simulink library "Diamond16AT_UNAL"  (Simulink 7.7)
settings: Solver=ode45  StartTime=0.0  StopTime=10.0  RelTol=1e-3
undefined symbols (not defined in the file or in its folder): Com1, none
libraries: xpcseriallib x2, Diamond16AT_UNAL x2
settings Model: Creator=BolivarNieto  LastModifiedBy=Edgar

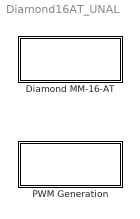
== system Diamond16AT_UNAL ==
  Diamond MM-16-AT : Subsystem
      mask Display: disp('Diamond MM-16-AT')
  PWM Generation : Subsystem
      mask Display: disp('PWM Generation')

== system Diamond16AT_UNAL/Diamond MM-16-AT ==
  MM-16-AT Analog Input : S-Function  FunctionName=addiamondmm16atcustom  Parameters=firstChan, numChans, range, sampleTime, baseDec  EnableBusSupport=off  mask{configuration=16 Single-ended, firstChan=1, numChans=12, range=0 to 5V, sampleTime=0.001, base=300}
      mask prompts: configuration "A/D Configuration"; firstChan "First channel: (From 1 to 8 or 16)"; numChans "Number of channels:"; sampleTime "Sample time:"; base "Base address (HEX):"
      mask help:
      | MM-16-AT
      | Diamond
      | Analog Input
      mask init:
      | phase = 2;
      | [baseDec, maskDisplay, maskDescription] = maskdiamondmm16(phase, configuration, firstChan, numChans, range, base);
      | set_param(gcb, 'MaskDescription', maskDescription);
      | set_param(gcb, 'MaskDisplay', maskDisplay);
      mask StyleString: popup(16 Single-ended|8   Differential inputs),edit,edit,popup(-10V to +10 V|-5V to +5V|-2.5V to +2.5V|-1.25V to +1.25V|-0.625V to +0.625V|0 to 10V|0 to 5V|0 to 2.5V|0 to 1.25V),edit,popup(220 |240 |250 |260 |280 |290 |2A0 |2B0 |2C0 |2D0 |2E0 |300 |330 |340 |350 |360 |380 |390 |3A0 |3C0 |3E0)
      mask Display: disp('MM-16-AT\nDiamond\nAnalog Input'); port_label('output', 1, '1'); port_label('output', 2, '2'); port_label('output', 3, '3'); port_label('output', 4, '4'); port_label('output', 5, '5'); port_label('output', 6, '6'); port_label('output', 7, '7'); port_label('output', 8, '8'); port_label('output', 9, '9'); port_label('output', 10, '10'); port_label('output', 11, '11'); port_label('output', 12, '12');
  MM-16-AT Analog Output : S-Function  FunctionName=dadiamondmm16at_custom  Parameters=channel, range, finalvalue, initValue, sampletime, basedec  EnableBusSupport=off  mask{channel=[ 1 2 3 4], range=0V to 5V, finalValuePop=Set all outputs to 0V, initValue=[0], sampletime=0.001, baseAddress=300}
      mask prompts: channel "Channel vector:"; range "Range vector"; finalValuePop "Behavior at model termination"; initValue "Initial value vector:"; sampletime "Sample time:"; baseAddress "Base address (HEX)"
      mask help:
      | MM-16-AT
      | Diamond Systems
      | Analog Output
      mask init:
      | boardType=1;
      | [maskdisplay, maskdescription, finalvalue, initValue, basedec] = mdadiamondmm16at_custom( boardType, channel, baseAddress, finalValuePop, initValue);
      | set_param(gcb,'MaskDescription',maskdescription);
      | set_param(gcb,'MaskDisplay',maskdisplay);
      mask StyleString: edit,popup(0V to 5V|-5V to 5V),popup(Set all outputs to 0V|Set to last value attained while the model was running),edit,edit,popup(220 |240 |250 |260 |280 |290 |2A0 |2B0 |2C0 |2D0 |2E0 |300 |330 |340 |350 |360 |380 |390 |3A0 |3C0 |3E0)
      mask Display: disp('MM-16-AT\nDiamond\nAnalog Output');port_label('input',1,'1');port_label('input',2,'2');port_label('input',3,'3');port_label('input',4,'4');
  MM-16-AT Digital Output : S-Function  FunctionName=dodiamond16at_custom  Parameters=channel, reset, initValue, sampleTime, basedec  EnableBusSupport=off  mask{channel=[1 2 3 4 5 6 7 8], reset=[0], initValue=[0], sampleTime=0.001, baseAddress2=300}
      mask prompts: channel "Channel vector:"; reset "Reset vector: (0 Hold last value, 1 set to initial value)"; initValue "Initial value vector:"; sampleTime "Sample Time:"; baseAddress2 "Base address (HEX):"
      mask help:
      | MM-16-AT
      | Diamond
      | Digital Output
      mask init:
      | deviceName = 'MM-16-AT';
      | [basedec, maskDisplay, maskDescription, reset, initValue] = mdodiamond16at_custom(deviceName, channel, sampleTime, baseAddress2, reset, initValue);
      | set_param(gcb, 'MaskDisplay', maskDisplay);
      | set_param(gcb, 'MaskDescription', maskDescription);
      mask StyleString: edit,edit,edit,edit,popup(220 |240 |250 |260 |280 |290 |2A0 |2B0 |2C0 |2D0 |2E0 |300 |330 |340 |350 |360 |380 |390 |3A0 |3C0 |3E0)
      mask Display: disp('MM-16-AT\nDiamond\nDigital Output'); port_label('input', 1, '1'); port_label('input', 2, '2'); port_label('input', 3, '3'); port_label('input', 4, '4'); port_label('input', 5, '5'); port_label('input', 6, '6'); port_label('input', 7, '7'); port_label('input', 8, '8');

== system Diamond16AT_UNAL/PWM Generation ==
  Motors - F4  STM - PWM : Subsystem  mask(Protocol for PWM generation through STM-F4){Satura=80, SamTime=0.001}
      mask prompts: Satura "Saturation (%):"; SamTime "Sample Time (s):"
      mask help:
      | Comunication protocol for PWM generation. This block communicates a STM-F4 through serial RS-232 comunication. The STM-F4 generates the PWMs required for motor control.
      |
      | INPUT:  [6x1] Percentage of duty cycle for each of the six motors.
      | OUTPUT: PWM signal to the H-Bridge
      mask Help:
      | Comunication protocol for PWM generation. This block communicates a STM-F4 through serial RS-232 comunication. The STM-F4 generates the PWMs required for motor control.
      | 
      | INPUT:  [6x1] Percentage of duty cycle for each of the six motors.
      | OUTPUT: PWM signal to the H-Bridge
  SG - Digital IO PWM Generation : Subsystem  mask(Stewart Gough Motors Block  ){PWM_amp=4, PWM_freq=1000, Rpm2Pwm=1, SampleTime_ed=0.001}
      mask prompts: PWM_amp "PWM Amplitude"; PWM_freq "PWM frequency (Hz)"; Rpm2Pwm "RPM to PWM's duty cycle gain"; SampleTime_ed "SampleTime"
      mask help: PWM Generator for 6 motors at the Stewart Gough. PWM generation is compatible with the H-Bridge 33887
      mask Help:
      | Set PWM parameters from the block dialog:
      | 
      | * PWM Amplitude stands for the amplitude when PWM is at high.
      | * RPM to PWM's duty cycle sets the conversion gain between the motor speed in RPM and the correspond duty cycle at the PWM generation.

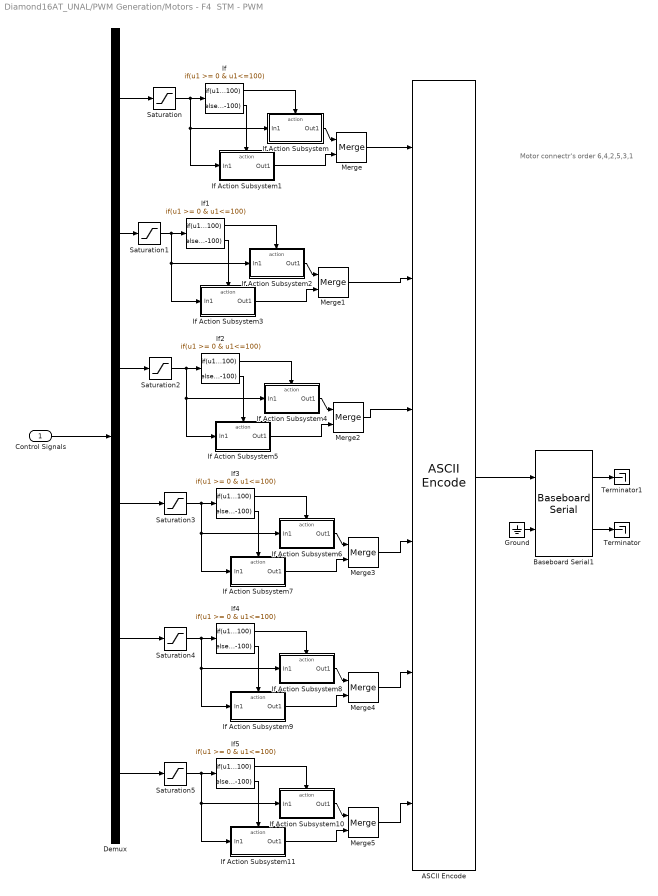
== system Diamond16AT_UNAL/PWM Generation/Motors - F4  STM - PWM ==
  note: Motor connectr's order 6,4,2,5,3,1
  Control Signals : Inport
  "ASCII Encode " : xpcseriallib/ASCII Encode   format=s%c%c%c%c%c%c  nvars=6  maxlength=9  vartypes={ 'double' }
  Baseboard Serial1 : xpcseriallib/Mainboard/Baseboard Serial  SystemSampleTime=-1  group=Board Setup  port=1  irqnum=4  saddr1=0x3f8  saddr2=0x3e8  config=Com1/none  baud1=115200  parity1=None  ndata1=8  nstop1=1  fifomode1=16 deep  rlevel1=half full  automode1=off  xmtfifosize1=1024  xmtdatatype1=8 bit uint null terminated  rcvfifosize1=1024  rcvmaxread1=1024  rcvminread1=1  rcvusedelim1=on  rcvdelim1=13  rcvdatatype1=count+16 bit uint  rcvsampletime1=.001  baud2=115200  parity2=None  ndata2=8  nstop2=1  fifomode2=16 deep  rlevel2=half full  automode2=off  xmtfifosize2=1024  xmtdatatype2=8 bit uint null terminated  rcvfifosize2=1024  rcvmaxread2=1024  rcvminread2=1  rcvusedelim2=on  rcvdelim2=13  rcvdatatype2=count+16 bit uint  rcvsampletime2=.001
  Demux : Demux  Outputs=6
  Ground : Ground
  If{,1..5} (6 alike) : If  IfExpression=u1 >= 0 & u1<=100  ElseIfExpressions=u1 <0 & u1 >= -100  ShowElse=off
  If Action Subsystem : Subsystem  TreatAsAtomicUnit=on
  If Action Subsystem1 : Subsystem  TreatAsAtomicUnit=on
  If Action Subsystem10 : Subsystem  TreatAsAtomicUnit=on
  If Action Subsystem11 : Subsystem  TreatAsAtomicUnit=on
  If Action Subsystem2 : Subsystem  TreatAsAtomicUnit=on
  If Action Subsystem3 : Subsystem  TreatAsAtomicUnit=on
  If Action Subsystem4 : Subsystem  TreatAsAtomicUnit=on
  If Action Subsystem5 : Subsystem  TreatAsAtomicUnit=on
  If Action Subsystem6 : Subsystem  TreatAsAtomicUnit=on
  If Action Subsystem7 : Subsystem  TreatAsAtomicUnit=on
  If Action Subsystem8 : Subsystem  TreatAsAtomicUnit=on
  If Action Subsystem9 : Subsystem  TreatAsAtomicUnit=on
  Merge{,1..5} (6 alike) : Merge
  Saturation{,1..5} (6 alike) : Saturate  UpperLimit=Satura  LowerLimit=-Satura  SampleTime=SamTime
  Terminator : Terminator
  Terminator1 : Terminator
  wires:
  "ASCII Encode "/1 -> Baseboard Serial1/1
  Baseboard Serial1/2 -> Terminator/1
  Baseboard Serial1/1 -> Terminator1/1
  Ground/1 -> Baseboard Serial1/2
  Control Signals/1 -> Demux/1
  If/1 -> If Action Subsystem/Action
  If/2 -> If Action Subsystem1/Action
  If Action Subsystem1/1(Out1) -> Merge/2
  If Action Subsystem/1(Out1) -> Merge/1
  Merge/1 -> "ASCII Encode "/1
  Saturation/1 -> If/1, If Action Subsystem/1(In1), If Action Subsystem1/1(In1)
  If1/1 -> If Action Subsystem2/Action
  If1/2 -> If Action Subsystem3/Action
  If Action Subsystem3/1(Out1) -> Merge1/2
  If Action Subsystem2/1(Out1) -> Merge1/1
  Saturation1/1 -> If1/1, If Action Subsystem2/1(In1), If Action Subsystem3/1(In1)
  If2/1 -> If Action Subsystem4/Action
  If2/2 -> If Action Subsystem5/Action
  If Action Subsystem5/1(Out1) -> Merge2/2
  If Action Subsystem4/1(Out1) -> Merge2/1
  Saturation2/1 -> If2/1, If Action Subsystem4/1(In1), If Action Subsystem5/1(In1)
  If3/1 -> If Action Subsystem6/Action
  If3/2 -> If Action Subsystem7/Action
  If Action Subsystem7/1(Out1) -> Merge3/2
  If Action Subsystem6/1(Out1) -> Merge3/1
  Saturation3/1 -> If3/1, If Action Subsystem6/1(In1), If Action Subsystem7/1(In1)
  If4/1 -> If Action Subsystem8/Action
  If4/2 -> If Action Subsystem9/Action
  If Action Subsystem9/1(Out1) -> Merge4/2
  If Action Subsystem8/1(Out1) -> Merge4/1
  Saturation4/1 -> If4/1, If Action Subsystem8/1(In1), If Action Subsystem9/1(In1)
  If5/1 -> If Action Subsystem10/Action
  If5/2 -> If Action Subsystem11/Action
  If Action Subsystem11/1(Out1) -> Merge5/2
  If Action Subsystem10/1(Out1) -> Merge5/1
  Saturation5/1 -> If5/1, If Action Subsystem10/1(In1), If Action Subsystem11/1(In1)
  Merge1/1 -> "ASCII Encode "/2
  Merge2/1 -> "ASCII Encode "/3
  Merge3/1 -> "ASCII Encode "/4
  Merge4/1 -> "ASCII Encode "/5
  Merge5/1 -> "ASCII Encode "/6
  Demux/1 -> Saturation/1
  Demux/2 -> Saturation1/1
  Demux/3 -> Saturation2/1
  Demux/4 -> Saturation3/1
  Demux/5 -> Saturation4/1
  Demux/6 -> Saturation5/1

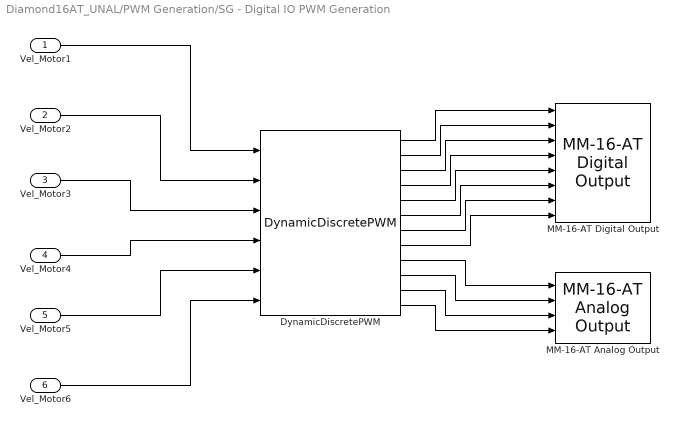
== system Diamond16AT_UNAL/PWM Generation/SG - Digital IO PWM Generation ==
  Vel_Motor1 : Inport
  Vel_Motor2 : Inport  Port=2
  Vel_Motor3 : Inport  Port=3
  Vel_Motor4 : Inport  Port=4
  Vel_Motor5 : Inport  Port=5
  Vel_Motor6 : Inport  Port=6
  DynamicDiscretePWM : S-Function  FunctionName=DynamicDiscretePWM  Parameters=Sample_Time,PWM_Amp,PWM_perio_Sample  EnableBusSupport=off  mask{PWM_perio=PWM_freq, PWM_Amp=PWM_amp, Sample_Time=SampleTime_ed}
      mask prompts: PWM_perio "PWM frequency (Hz)"; PWM_Amp "PWM Amplitude"; Sample_Time "Sample Time (s)"
      mask init:
      | PWM_perio_Sample=1/PWM_perio;
      | PWM_perio_Sample=round(PWM_perio_Sample/Sample_Time);
  MM-16-AT Analog Output : Diamond16AT_UNAL/Diamond MM-16-AT/MM-16-AT Analog Output  channel=[ 1 2 3 4]  range=0V to 5V  finalValuePop=Set all outputs to 0V  initValue=[0]  sampletime=SampleTime_ed  baseAddress=300
  MM-16-AT Digital Output : Diamond16AT_UNAL/Diamond MM-16-AT/MM-16-AT Digital Output  channel=[1 2 3 4 5 6 7 8]  reset=[1]  initValue=[0]  sampleTime=SampleTime_ed  baseAddress2=300
  wires:
  DynamicDiscretePWM/1 -> MM-16-AT Digital Output/1
  DynamicDiscretePWM/2 -> MM-16-AT Digital Output/2
  DynamicDiscretePWM/3 -> MM-16-AT Digital Output/3
  DynamicDiscretePWM/4 -> MM-16-AT Digital Output/4
  DynamicDiscretePWM/5 -> MM-16-AT Digital Output/5
  DynamicDiscretePWM/6 -> MM-16-AT Digital Output/6
  DynamicDiscretePWM/7 -> MM-16-AT Digital Output/7
  DynamicDiscretePWM/8 -> MM-16-AT Digital Output/8
  DynamicDiscretePWM/9 -> MM-16-AT Analog Output/1
  DynamicDiscretePWM/10 -> MM-16-AT Analog Output/2
  DynamicDiscretePWM/11 -> MM-16-AT Analog Output/3
  DynamicDiscretePWM/12 -> MM-16-AT Analog Output/4
  Vel_Motor1/1 -> DynamicDiscretePWM/1
  Vel_Motor2/1 -> DynamicDiscretePWM/2
  Vel_Motor3/1 -> DynamicDiscretePWM/3
  Vel_Motor4/1 -> DynamicDiscretePWM/4
  Vel_Motor5/1 -> DynamicDiscretePWM/5
  Vel_Motor6/1 -> DynamicDiscretePWM/6

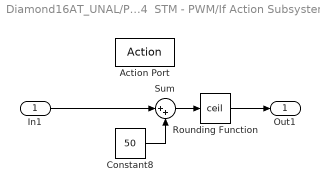
== system Diamond16AT_UNAL/PWM Generation/Motors - F4  STM - PWM/If Action Subsystem ==
  In1 : Inport
  Action Port : ActionPort
  Constant8 : Constant  Value=50
  Rounding Function : Rounding  Operator=ceil
  Sum : Sum  Inputs=|++
  Out1 : Outport
  wires:
  In1/1 -> Sum/1
  Sum/1 -> Rounding Function/1
  Constant8/1 -> Sum/2
  Rounding Function/1 -> Out1/1

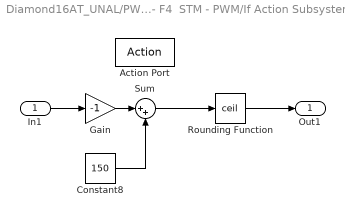
== system Diamond16AT_UNAL/PWM Generation/Motors - F4  STM - PWM/If Action Subsystem1 ==
  In1 : Inport
  Action Port : ActionPort
  Constant8 : Constant  Value=150
  Gain : Gain  Gain=-1
  Rounding Function : Rounding  Operator=ceil
  Sum : Sum  Inputs=|++
  Out1 : Outport
  wires:
  In1/1 -> Gain/1
  Gain/1 -> Sum/1
  Constant8/1 -> Sum/2
  Sum/1 -> Rounding Function/1
  Rounding Function/1 -> Out1/1

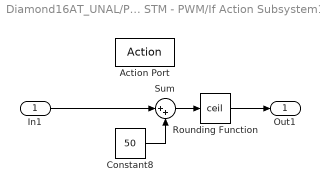
== system Diamond16AT_UNAL/PWM Generation/Motors - F4  STM - PWM/If Action Subsystem10 ==
  In1 : Inport
  Action Port : ActionPort
  Constant8 : Constant  Value=50
  Rounding Function : Rounding  Operator=ceil
  Sum : Sum  Inputs=|++
  Out1 : Outport
  wires:
  In1/1 -> Sum/1
  Sum/1 -> Rounding Function/1
  Constant8/1 -> Sum/2
  Rounding Function/1 -> Out1/1

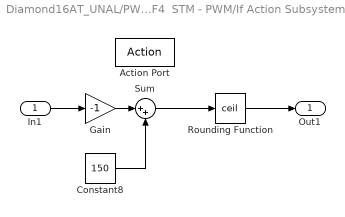
== system Diamond16AT_UNAL/PWM Generation/Motors - F4  STM - PWM/If Action Subsystem11 ==
  In1 : Inport
  Action Port : ActionPort
  Constant8 : Constant  Value=150
  Gain : Gain  Gain=-1
  Rounding Function : Rounding  Operator=ceil
  Sum : Sum  Inputs=|++
  Out1 : Outport
  wires:
  In1/1 -> Gain/1
  Gain/1 -> Sum/1
  Constant8/1 -> Sum/2
  Sum/1 -> Rounding Function/1
  Rounding Function/1 -> Out1/1

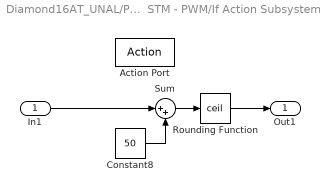
== system Diamond16AT_UNAL/PWM Generation/Motors - F4  STM - PWM/If Action Subsystem2 ==
  In1 : Inport
  Action Port : ActionPort
  Constant8 : Constant  Value=50
  Rounding Function : Rounding  Operator=ceil
  Sum : Sum  Inputs=|++
  Out1 : Outport
  wires:
  In1/1 -> Sum/1
  Sum/1 -> Rounding Function/1
  Constant8/1 -> Sum/2
  Rounding Function/1 -> Out1/1

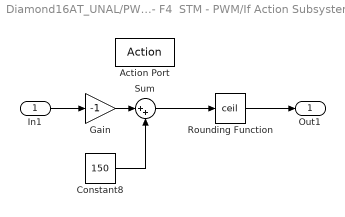
== system Diamond16AT_UNAL/PWM Generation/Motors - F4  STM - PWM/If Action Subsystem3 ==
  In1 : Inport
  Action Port : ActionPort
  Constant8 : Constant  Value=150
  Gain : Gain  Gain=-1
  Rounding Function : Rounding  Operator=ceil
  Sum : Sum  Inputs=|++
  Out1 : Outport
  wires:
  In1/1 -> Gain/1
  Gain/1 -> Sum/1
  Constant8/1 -> Sum/2
  Sum/1 -> Rounding Function/1
  Rounding Function/1 -> Out1/1

== system Diamond16AT_UNAL/PWM Generation/Motors - F4  STM - PWM/If Action Subsystem4 ==
  In1 : Inport
  Action Port : ActionPort
  Constant8 : Constant  Value=50
  Rounding Function : Rounding  Operator=ceil
  Sum : Sum  Inputs=|++
  Out1 : Outport
  wires:
  In1/1 -> Sum/1
  Sum/1 -> Rounding Function/1
  Constant8/1 -> Sum/2
  Rounding Function/1 -> Out1/1

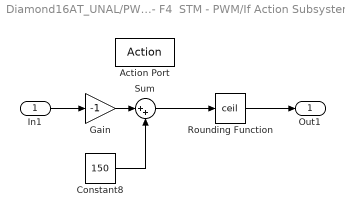
== system Diamond16AT_UNAL/PWM Generation/Motors - F4  STM - PWM/If Action Subsystem5 ==
  In1 : Inport
  Action Port : ActionPort
  Constant8 : Constant  Value=150
  Gain : Gain  Gain=-1
  Rounding Function : Rounding  Operator=ceil
  Sum : Sum  Inputs=|++
  Out1 : Outport
  wires:
  In1/1 -> Gain/1
  Gain/1 -> Sum/1
  Constant8/1 -> Sum/2
  Sum/1 -> Rounding Function/1
  Rounding Function/1 -> Out1/1

== system Diamond16AT_UNAL/PWM Generation/Motors - F4  STM - PWM/If Action Subsystem6 ==
  In1 : Inport
  Action Port : ActionPort
  Constant8 : Constant  Value=50
  Rounding Function : Rounding  Operator=ceil
  Sum : Sum  Inputs=|++
  Out1 : Outport
  wires:
  In1/1 -> Sum/1
  Sum/1 -> Rounding Function/1
  Constant8/1 -> Sum/2
  Rounding Function/1 -> Out1/1

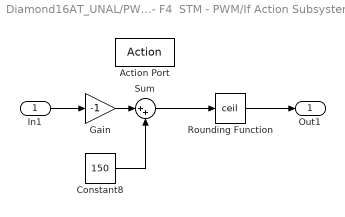
== system Diamond16AT_UNAL/PWM Generation/Motors - F4  STM - PWM/If Action Subsystem7 ==
  In1 : Inport
  Action Port : ActionPort
  Constant8 : Constant  Value=150
  Gain : Gain  Gain=-1
  Rounding Function : Rounding  Operator=ceil
  Sum : Sum  Inputs=|++
  Out1 : Outport
  wires:
  In1/1 -> Gain/1
  Gain/1 -> Sum/1
  Constant8/1 -> Sum/2
  Sum/1 -> Rounding Function/1
  Rounding Function/1 -> Out1/1

== system Diamond16AT_UNAL/PWM Generation/Motors - F4  STM - PWM/If Action Subsystem8 ==
  In1 : Inport
  Action Port : ActionPort
  Constant8 : Constant  Value=50
  Rounding Function : Rounding  Operator=ceil
  Sum : Sum  Inputs=|++
  Out1 : Outport
  wires:
  In1/1 -> Sum/1
  Sum/1 -> Rounding Function/1
  Constant8/1 -> Sum/2
  Rounding Function/1 -> Out1/1

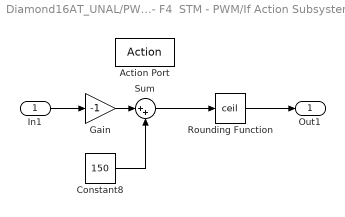
== system Diamond16AT_UNAL/PWM Generation/Motors - F4  STM - PWM/If Action Subsystem9 ==
  In1 : Inport
  Action Port : ActionPort
  Constant8 : Constant  Value=150
  Gain : Gain  Gain=-1
  Rounding Function : Rounding  Operator=ceil
  Sum : Sum  Inputs=|++
  Out1 : Outport
  wires:
  In1/1 -> Gain/1
  Gain/1 -> Sum/1
  Constant8/1 -> Sum/2
  Sum/1 -> Rounding Function/1
  Rounding Function/1 -> Out1/1
